simulink model "controlblackboxTrajectory"  (R2019a)
settings: Solver=VariableStepAuto  StartTime=0.0  StopTime=10.0  RelTol=1e-3
libraries: simulink x1
settings Model: Creator=joseluis.martin  LastModifiedBy=joseluis.martin

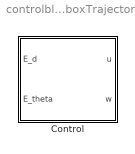
== system controlblackboxTrajectory ==
  Control : Subsystem

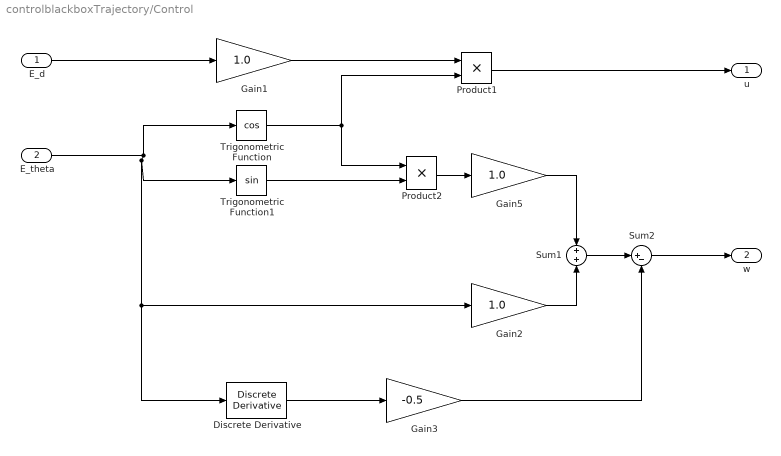
== system controlblackboxTrajectory/Control ==
  E_d : Inport
  E_theta : Inport  Port=2
  Discrete Derivative : simulink/Discrete/Discrete Derivative  gainval=1.0  ICPrevScaledInput=0.0  OutMin=[]  OutMax=[]  OutDataType=fixdt(1, 16)  OutScaling=2^-10  DoSatur=off
  Gain1 : Gain  Gain=1.0
  Gain2 : Gain  Gain=1.0
  Gain3 : Gain  Gain=-0.5
  Gain5 : Gain  Gain=1.0
  Product1 : Product
  Product2 : Product
  Sum1 : Sum
  Sum2 : Sum  Inputs=|+-
  Trigonometric Function : Trigonometry  Operator=cos
  Trigonometric Function1 : Trigonometry
  u : Outport
  w : Outport  Port=2
  wires:
  E_theta/1 -> Trigonometric Function/1, Trigonometric Function1/1, Discrete Derivative/1, Gain2/1
  E_d/1 -> Gain1/1
  Trigonometric Function/1 -> Product1/2, Product2/1
  Trigonometric Function1/1 -> Product2/2
  Product2/1 -> Gain5/1
  Gain1/1 -> Product1/1
  Gain5/1 -> Sum1/1
  Gain2/1 -> Sum1/2
  Product1/1 -> u/1
  Sum1/1 -> Sum2/1
  Sum2/1 -> w/1
  Discrete Derivative/1 -> Gain3/1
  Gain3/1 -> Sum2/2
